simulink model "mModelWorkspaceCopy"  (R2012b)
settings: Solver=FixedStepDiscrete  StartTime=0.0  StopTime=10.0  RelTol=1e-3
undefined symbols (not defined in the file or in its folder): k, k1, k2, k3
CloseFcn:
  | rtwprivate ssgencode ModelCloseRequest prob1
settings Model: ExtModeAutoUpdateStatusClock=off  Creator=stoeppe  LastModifiedBy=hungdang
settings DataIOCC: SaveFormat=StructureWithTime  SignalLoggingSaveFormat=ModelDataLogs  SignalLoggingName=sigsOut
settings OptimizationCC: InlineParams=on  InitFltsAndDblsToZero=on  OptimizeModelRefInitCode=on  LifeSpan=1
settings DebuggingCC: SaveWithParameterizedLinksMsg=none  SolverPrmCheckMsg=none  MultiTaskDSMMsg=warning  MultiTaskCondExecSysMsg=none  FcnCallInpInsideContextMsg=UseLocalSettings
settings HardwareCC: TargetUnknown=on
settings RTWCC: SystemTargetFile=ert.tlc  GenCodeOnly=on  TemplateMakefile=ert_default_tmf  GenerateReport=on  ProcessScript=ert_make_rtw_hook  IncludeHyperlinkInReport=on  LaunchReport=on  IncludeERTFirstTime=on
settings CodeAppCC: IgnoreCustomStorageClasses=off
settings ERTTargetCC: TargetFcnLib=ansi_tfl_tmw.mat  CodeReplacementLibrary=ANSI_C  MultiwordLength=2048  GenerateSampleERTMain=on  InlinedParameterPlacement=NonHierarchical  ERTCustomFileTemplate=example_file_process.tlc  ConvertIfToSwitch=off  SuppressUnreachableDefaultCases=off

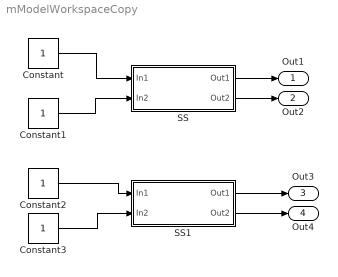
== system mModelWorkspaceCopy ==
  Constant{,1..3} (4 alike) : Constant  SampleTime=1
  SS : Subsystem  TreatAsAtomicUnit=on
  SS1 : Subsystem  TreatAsAtomicUnit=on
  Out1 : Outport
  Out2 : Outport  Port=2
  Out3 : Outport  Port=3
  Out4 : Outport  Port=4
  wires:
  Constant/1 -> SS/1(In1)
  SS/1(Out1) -> Out1/1
  SS/2(Out2) -> Out2/1
  Constant1/1 -> SS/2(In2)
  Constant2/1 -> SS1/1(In1)
  Constant3/1 -> SS1/2(In2)
  SS1/1(Out1) -> Out3/1
  SS1/2(Out2) -> Out4/1

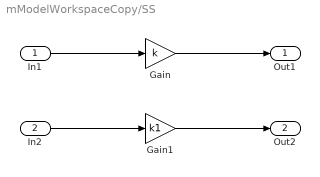
== system mModelWorkspaceCopy/SS ==
  In1 : Inport
  In2 : Inport  Port=2
  Gain : Gain  Gain=k
  Gain1 : Gain  Gain=k1
  Out1 : Outport
  Out2 : Outport  Port=2
  wires:
  In1/1 -> Gain/1
  Gain/1 -> Out1/1
  In2/1 -> Gain1/1
  Gain1/1 -> Out2/1

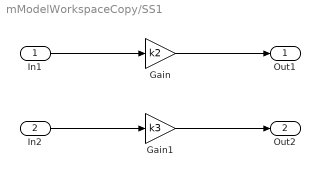
== system mModelWorkspaceCopy/SS1 ==
  In1 : Inport
  In2 : Inport  Port=2
  Gain : Gain  Gain=k2
  Gain1 : Gain  Gain=k3
  Out1 : Outport
  Out2 : Outport  Port=2
  wires:
  In1/1 -> Gain/1
  Gain/1 -> Out1/1
  In2/1 -> Gain1/1
  Gain1/1 -> Out2/1
